simulink model "System1"  (R2019a)
settings: Solver=ode4  StartTime=0.0  StopTime=2.0  FixedStep=0.05  RelTol=1e-3
settings Model: Creator=vmali  LastModifiedBy=vmali

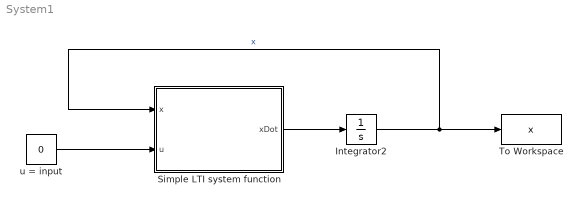
== system System1 ==
  Integrator2 : Integrator  InitialCondition=2.0
  Simple LTI system function : MATLAB Function  TreatAsAtomicUnit=on
  To Workspace : ToWorkspace  VariableName=x  SaveFormat=Timeseries  SampleTime=-1
  u = input : Constant  Value=0
  wires:
  Simple LTI system function/1(xDot) -> Integrator2/1
  Integrator2/1 -> To Workspace/1, Simple LTI system function/1(x)  "x"
  u = input/1 -> Simple LTI system function/2(u)

== matlab function System1/Simple LTI system function ==
  data: x input; u input; xDot output
function xDot = f(x,u)

% fill in f of x' = f(x,u)
xDot = -4*x + u ;
